simulink model "figure9"  (R2015b)
settings: Solver=FixedStepAuto  StartTime=0.0  StopTime=2  RelTol=1e-3
values from neighbouring files (symbols this model uses):
  bHI = 35    [Initiation.m]
  bWall = 0    [Initiation.m]    (also in VirtualEnvironment.m = block.DialogPrm(2).Data; Virtual_Environment.m = block.DialogPrm(2).Data)
  kWall = 90000    [Initiation.m]    (also in VirtualEnvironment.m = block.DialogPrm(1).Data; Virtual_Environment.m = block.DialogPrm(1).Data)
  m = 1    [Initiation.m]
  nWall = 1    [Initiation.m]    (also in VirtualEnvironment.m = block.DialogPrm(3).Data; Virtual_Environment.m = block.DialogPrm(3).Data)
  tsampling = 0.001    [Initiation.m]    (also in VirtualEnvironment.m = block.DialogPrm(6).Data; Virtual_Environment.m = block.DialogPrm(6).Data)
  x0 = 0.14    [Initiation.m]    (also in PC.m = []; Wall.m = []; devision.m = []; sgn.m = [])
  x_dot0 = 0    [Initiation.m]
  xWall = 0.085    [Initiation.m]
libraries: simulink x3
settings Model: Creator=TOSHIBA  LastModifiedBy=TOSHIBA

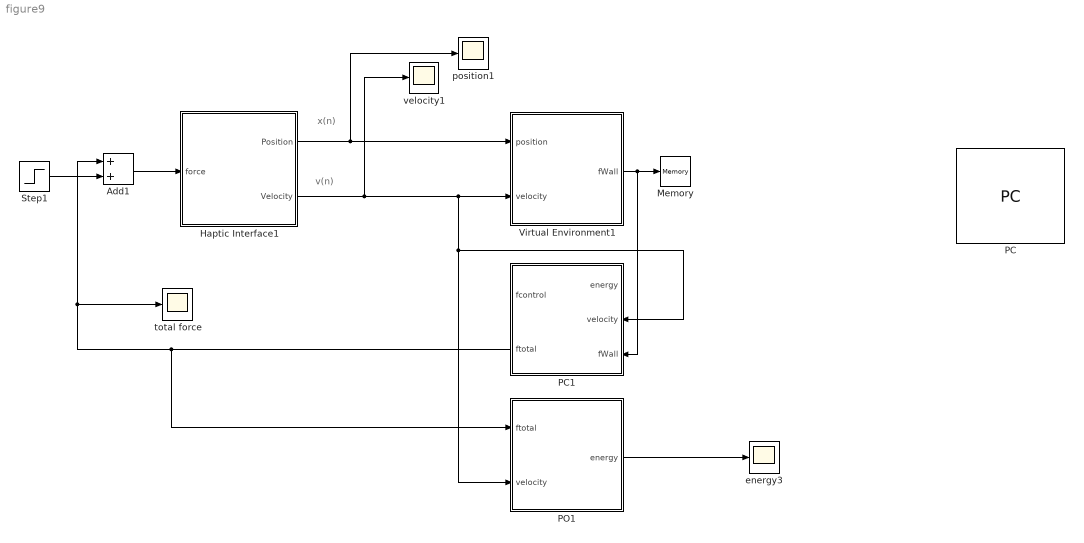
== system figure9 ==
  note: v(n)
  note: x(n)
  Add1 : Sum
  Haptic Interface1 : Subsystem
  Memory : Memory
  PC : S-Function  FunctionName=PC  Parameters=tsampling,tsampling  SFunctionDeploymentMode=off  EnableBusSupport=off
  PC1 : Subsystem
  PO1 : Subsystem
  Step1 : Step  Time=0.3  After=-10  SampleTime=0
  Virtual Environment1 : Subsystem
  energy3 : Scope
  position1 : Scope
  total force : Scope
  velocity1 : Scope
  wires:
  Haptic Interface1/1(Position) -> position1/1, Virtual Environment1/1(position)
  Add1/1 -> Haptic Interface1/1(force)
  Step1/1 -> Add1/2
  Haptic Interface1/2(Velocity) -> PO1/2(velocity), PC1/2(velocity), Virtual Environment1/2(velocity), velocity1/1
  PO1/1(energy) -> energy3/1
  PC1/2(ftotal) -> Add1/1, total force/1, PO1/1(ftotal)
  Virtual Environment1/1(fWall) -> PC1/3(fWall), Memory/1

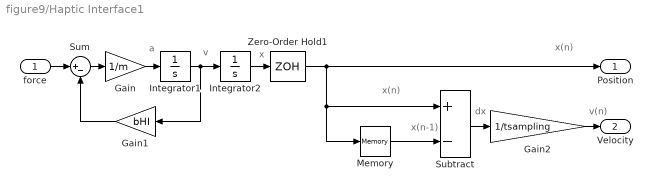
== system figure9/Haptic Interface1 ==
  note: v(n)
  note: dx
  note: x(n-1)
  note: x(n)
  note: x(n)
  note: x
  note: v
  note: a
  force : Inport
  Gain : Gain  Gain=1/m
  Gain1 : Gain  Gain=bHI
  Gain2 : Gain  Gain=1/tsampling
  Integrator1 : Integrator  InitialCondition=x_dot0
  Integrator2 : Integrator  InitialCondition=x0
  Memory : Memory  X0=x0
  Subtract : Sum  Inputs=+-
  Sum : Sum  Inputs=|+-
  Zero-Order Hold1 : ZeroOrderHold  SampleTime=tsampling
  Position : Outport
  Velocity : Outport  Port=2
  wires:
  Gain2/1 -> Velocity/1
  Subtract/1 -> Gain2/1
  Memory/1 -> Subtract/2
  Integrator2/1 -> Zero-Order Hold1/1
  Integrator1/1 -> Gain1/1, Integrator2/1
  Gain/1 -> Integrator1/1
  force/1 -> Sum/1
  Sum/1 -> Gain/1
  Gain1/1 -> Sum/2
  Zero-Order Hold1/1 -> Memory/1, Subtract/1, Position/1

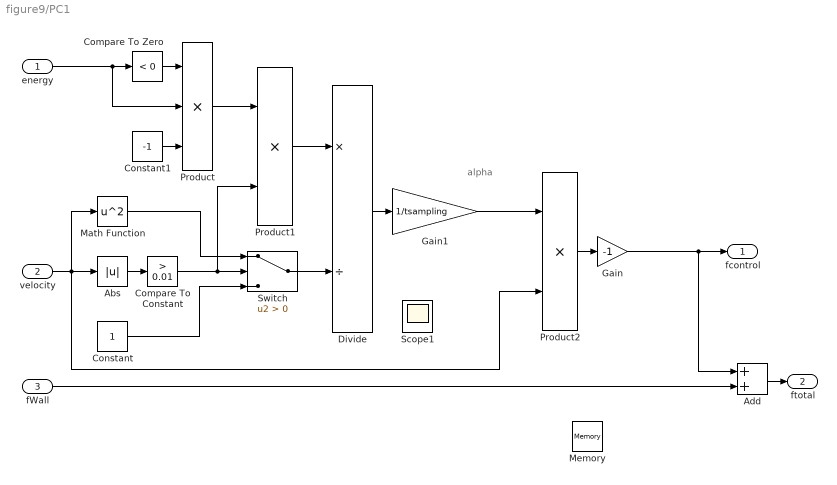
== system figure9/PC1 ==
  note: alpha
  energy : Inport
  velocity : Inport  Port=2
  fWall : Inport  Port=3
  Abs : Abs
  Add : Sum
  Compare To Constant : simulink/Logic and Bit Operations/Compare To Constant  relop=>  const=0.01  OutDataTypeStr=boolean
  Compare To Zero : simulink/Logic and Bit Operations/Compare To Zero  relop=<  OutDataTypeStr=boolean
  Constant : Constant
  Constant1 : Constant  Value=-1
  Divide : Product  Inputs=*/
  Gain : Gain  Gain=-1
  Gain1 : Gain  Gain=1/tsampling
  Math Function : Math  Operator=square  SaturateOnIntegerOverflow=on
  Memory : Memory
  Product : Product  Inputs=3
  Product1 : Product
  Product2 : Product
  Scope1 : Scope
  Switch : Switch  Criteria=u2 > Threshold
  fcontrol : Outport
  ftotal : Outport  Port=2
  wires:
  Compare To Zero/1 -> Product/1
  Compare To Constant/1 -> Switch/2, Product1/2
  Constant/1 -> Switch/3
  Math Function/1 -> Switch/1
  Gain1/1 -> Product2/1
  Divide/1 -> Gain1/1
  Product1/1 -> Divide/1
  Product2/1 -> Gain/1
  Switch/1 -> Divide/2
  Add/1 -> ftotal/1
  Product/1 -> Product1/1
  Constant1/1 -> Product/3
  Abs/1 -> Compare To Constant/1
  energy/1 -> Product/2, Compare To Zero/1
  velocity/1 -> Abs/1, Math Function/1, Product2/2
  Gain/1 -> fcontrol/1, Add/1
  fWall/1 -> Add/2

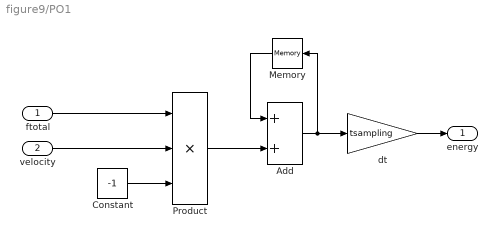
== system figure9/PO1 ==
  ftotal : Inport
  velocity : Inport  Port=2
  Add : Sum
  Constant : Constant  Value=-1
  Memory : Memory
  Product : Product  Inputs=3
  dt : Gain  Gain=tsampling
  energy : Outport
  wires:
  Add/1 -> dt/1, Memory/1
  Memory/1 -> Add/1
  Product/1 -> Add/2
  dt/1 -> energy/1
  Constant/1 -> Product/3
  velocity/1 -> Product/2
  ftotal/1 -> Product/1

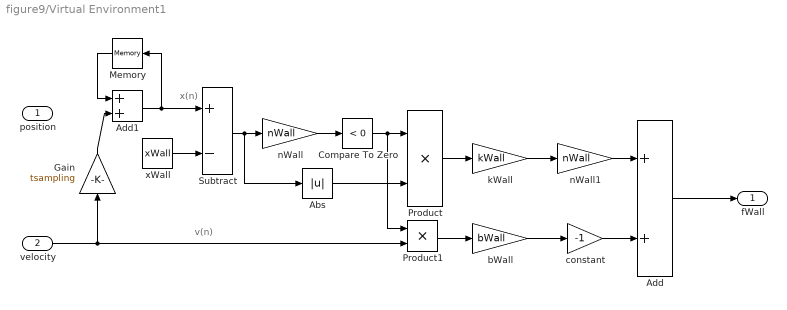
== system figure9/Virtual Environment1 ==
  note: v(n)
  note: x(n)
  position : Inport
  velocity : Inport  Port=2
  Abs : Abs
  Add : Sum
  Add1 : Sum
  Compare To Zero : simulink/Logic and Bit Operations/Compare To Zero  relop=<  OutDataTypeStr=boolean
  Gain : Gain  Gain=tsampling
  Memory : Memory  X0=x0
  Product : Product
  Product1 : Product
  Subtract : Sum  Inputs=+-
  bWall : Gain  Gain=bWall
  constant : Gain  Gain=-1
  kWall : Gain  Gain=kWall
  nWall : Gain  Gain=nWall
  nWall1 : Gain  Gain=nWall
  xWall : Constant  Value=xWall
  fWall : Outport
  wires:
  xWall/1 -> Subtract/2
  Subtract/1 -> Abs/1, nWall/1
  nWall/1 -> Compare To Zero/1
  Compare To Zero/1 -> Product1/1, Product/1
  Abs/1 -> Product/2
  Product/1 -> kWall/1
  kWall/1 -> nWall1/1
  bWall/1 -> constant/1
  constant/1 -> Add/2
  nWall1/1 -> Add/1
  Product1/1 -> bWall/1
  velocity/1 -> Gain/1, Product1/2
  Add1/1 -> Subtract/1, Memory/1
  Gain/1 -> Add1/2
  Memory/1 -> Add1/1
  Add/1 -> fWall/1
